simulink model "Rectifier"  (R2023b)
settings: Solver=VariableStepAuto  StartTime=0.0  StopTime=1  MaxStep=1e-4  RelTol=1e-4
values from neighbouring files (symbols this model uses):
  frequency_voltage1 = 60    [paramVals.mat]
  frequency_voltage2 = 60    [paramVals.mat]
  frequency_voltage3 = 60    [paramVals.mat]
  L = 0.2    [paramVals.mat]
  L1 = 0.005    [paramVals.mat]
  L2 = 0.005    [paramVals.mat]
  L3 = 0.005    [paramVals.mat]
  Load_Resistance_Ohm = 10    [paramVals.mat]
  peakAmplitude_voltage1 = 169.705627485    [paramVals.mat]
  peakAmplitude_voltage2 = 169.705627485    [paramVals.mat]
  peakAmplitude_voltage3 = 169.705627485    [paramVals.mat]
  phaseInDegree_voltage1 = 0    [paramVals.mat]
  phaseInDegree_voltage2 = -120    [paramVals.mat]
  phaseInDegree_voltage3 = 120    [paramVals.mat]
libraries: spsGroundLib x5, spsSeriesRLCBranchLib x5, spsDiodeLib x3, spsACVoltageSourceLib x3, spsCurrentMeasurementLib x1, spsVoltageMeasurementLib x1, spspowerguiLib x1
settings Model: Creator=The MathWorks, Inc.  LastModifiedBy=z004f2se
settings SolverCC: AlgebraicLoopSolver=TrustRegion
settings DataIOCC: ReturnWorkspaceOutputs=off  SignalLoggingName=sigsOut
settings OptimizationCC: BlockReduction=off  BooleanDataType=off  ExpressionDepthLimit=2147483647  InitFltsAndDblsToZero=on  EfficientMapNaN2IntZero=off  LifeSpan=inf
settings DebuggingCC: SaveWithParameterizedLinksMsg=none  UnderspecifiedInitializationDetection=Classic  MergeDetectMultiDrivingBlocksExec=none  CheckExecutionContextPreStartOutputMsg=on  SignalResolutionControl=TryResolveAllWithWarning  MultiTaskDSMMsg=warning  MultiTaskCondExecSysMsg=none  SigSpecEnsureSampleTimeMsg=none  FcnCallInpInsideContextMsg=warning  UnconnectedInputMsg=warning  UnconnectedOutputMsg=warning  UnconnectedLineMsg=warning  StateNameClashWarn=warning  SFUnexpectedBacktrackingDiag=warning  SFNoUnconditionalDefaultTransitionDiag=warning  SFExecutionAtInitializationDiag=none  ArithmeticOperatorsInVariantConditions=warning
settings HardwareCC: ProdBitPerPointer=32  ProdBitPerSizeT=32  ProdBitPerPtrDiffT=32  ProdLargestAtomicFloat=None  ProdIntDivRoundTo=Undefined  ProdEndianess=Unspecified  ProdWordSize=32  ProdHWDeviceType=32-bit Generic  TargetUnknown=on
settings ModelReferenceCC: EnableRefExpFcnMdlSchedulingChecks=on  PropagateSignalLabelsOutOfModel=off
settings SFSimCC: SimUseLocalCustomCode=off  CustomCodeUndefinedFunction=UseInterfaceOnly
settings RTWCC: RTWUseLocalCustomCode=off  DLArmComputeVersion=19.05
settings CodeAppCC: StateflowObjectComments=on
settings GRTTargetCC: TargetFcnLib=ansi_tfl_tmw.mat  TargetLangStandard=C89/C90 (ANSI)  CombineOutputUpdateFcns=off  GRTInterface=on
settings ConfigComp: CovMetricSettings=dw  CovSaveCumulativeToWorkspaceVar=on  CovSaveSingleToWorkspaceVar=on  CovExternalEMLEnable=off  CovSFcnEnable=off
settings SimscapeCC: SimscapeNormalizeSystem=off  SimscapeNominalValues={1, 'bar'; 1, 'cm^3/s'; 1, 'bar*kg/s'; 1, 'kJ/kg'; 1, 'kW'; }

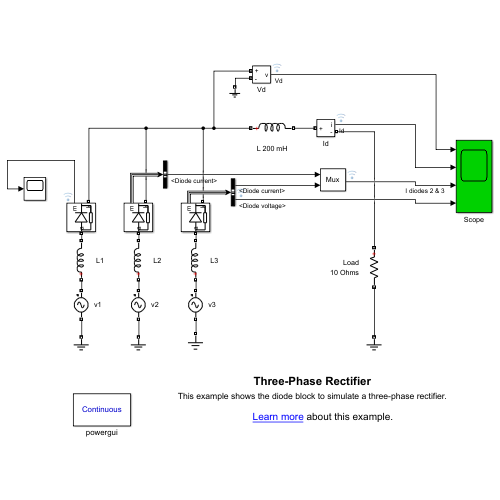
[thumbnail: Simulink's stored preview of the top-level diagram]
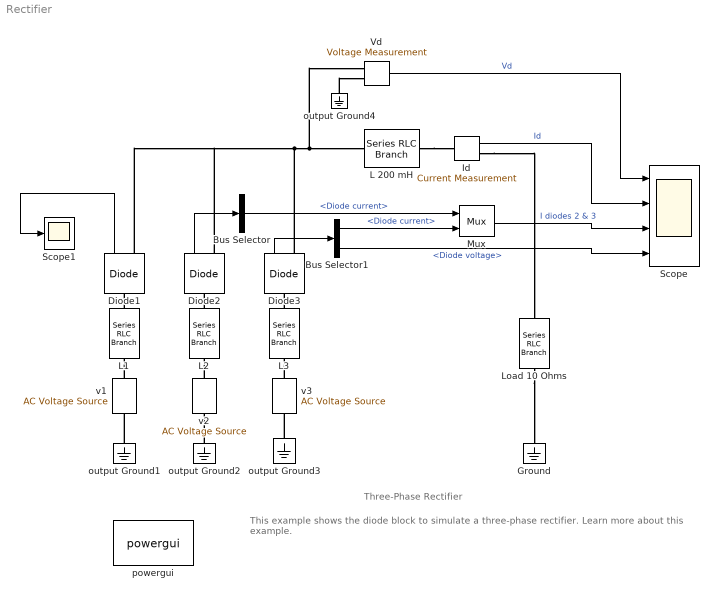
== system Rectifier ==
  note: Three-Phase Rectifier
  note: This example shows the diode block to simulate a three-phase rectifier.
      |
      | Learn more about this example.
  Bus Selector : BusSelector  OutputSignals=Diode current
  Bus Selector1 : BusSelector  OutputSignals=Diode current,Diode voltage
  Diode1 : spsDiodeLib/Diode  Ron=RonRes_Diode1  Lon=0  Vf=forwardVoltage_Diode1  IC=0  UseSnubber=off  Rs=snubberResmOhm_Diode1  Cs=snubberCapF_Diode1  Measurements=on
      settings: AttributesFormatString=\n
  Diode2 : spsDiodeLib/Diode  Ron=1e-2  Lon=0  Vf=0.8  IC=0  UseSnubber=off  Rs=1000  Cs=0.1e-6  Measurements=on
      settings: AttributesFormatString=\n
  Diode3 : spsDiodeLib/Diode  Ron=1e-2  Lon=0  Vf=0.8  IC=0  UseSnubber=off  Rs=1000  Cs=0.1e-6  Measurements=on
      settings: AttributesFormatString=\n
  Ground : spsGroundLib/Ground  LConnTagsString=a
  Id : spsCurrentMeasurementLib/Current Measurement  Tag=PoWeRsYsTeMmEaSuReMeNt  PhasorSimulation=off  OutputType=Magnitude  PSBequivalent=0
      settings: AttributesFormatString=\n
  L 200 mH : spsSeriesRLCBranchLib/Series RLC Branch  LConnTagsString=__new0  RConnTagsString=__new0  BranchType=L  Resistance=[]  Inductance=L  SetiL0=off  InitialCurrent=0  Capacitance=[]  Setx0=off  InitialVoltage=0  Measurements=None
  L1 : spsSeriesRLCBranchLib/Series RLC Branch  LConnTagsString=__new0  RConnTagsString=__new0  BranchType=L  Resistance=[]  Inductance=L1  SetiL0=off  InitialCurrent=0  Capacitance=[]  Setx0=off  InitialVoltage=0  Measurements=None
  L2 : spsSeriesRLCBranchLib/Series RLC Branch  LConnTagsString=__new0  RConnTagsString=__new0  BranchType=L  Resistance=[]  Inductance=L2  SetiL0=off  InitialCurrent=0  Capacitance=[]  Setx0=off  InitialVoltage=0  Measurements=None
  L3 : spsSeriesRLCBranchLib/Series RLC Branch  LConnTagsString=__new0  RConnTagsString=__new0  BranchType=L  Resistance=[]  Inductance=L3  SetiL0=off  InitialCurrent=0  Capacitance=[]  Setx0=off  InitialVoltage=0  Measurements=None
  Load 10 Ohms : spsSeriesRLCBranchLib/Series RLC Branch  LConnTagsString=__new0  RConnTagsString=__new0  BranchType=R  Resistance=Load_Resistance_Ohm  Inductance=[]  SetiL0=off  InitialCurrent=0  Capacitance=[]  Setx0=off  InitialVoltage=0  Measurements=None
  Mux : Mux  Inputs=2
  Scope : Scope  NumInputPorts=4
  Scope1 : Scope
  Vd : spsVoltageMeasurementLib/Voltage Measurement  Tag=PoWeRsYsTeMmEaSuReMeNt  PhasorSimulation=off  OutputType=Magnitude  PSBequivalent=0
  output Ground{1..4} (4 alike) : spsGroundLib/Ground  LConnTagsString=a
  powergui : spspowerguiLib/powergui  Priority=2  SimulationMode=Continuous  SampleTime=0  frequency=60  Iterations=50  frequencyindice=60  Pbase=100e6  ErrMax=1e-4  UnitsV=kV  UnitsW=MW  buscounter=0  FunctionMessages=off  echomessages=off  EnableUseOfTLC=off  CurrentSourceSwitches=off  DisableSnubberDevices=off  DisableRonSwitches=off  DisableVfSwitches=off  DisplayEquations=off  AutomaticDiscreteSolvers=off  SolverType=Tustin/Backward Euler (TBE)  Interpol=off  ExternalGateDelay=off  methode=off  Ts=100  x0status=blocks  SPID=on  SwTol=0  HookPort=off  NonlinearTolerance=1e-4  nMaxIteration=100  ContinueOnMaxIteration=off  RestoreLinks=warning  ResistiveCurrentMeasurement=off  Frange=[0:2:500]  Ylog=off  Xlog=on  ShowGrid=off  save=off  variable=ZData  structure=0  ZoomFFT=on  StartTime=0.0  cycles=1  DisplayStyle=1  fundamental=60  FreqAxis=off  MaxFrequency=1000  frequencyindicesteady=1  RmsSteady=1  display=off
  v1 : spsACVoltageSourceLib/AC Voltage Source  Description=source block  Amplitude=peakAmplitude_voltage1  Phase=phaseInDegree_voltage1  Frequency=frequency_voltage1  SampleTime=0  Measurements=None  BusType=swing  Pref=10e3  Qref=0  Qmin=-inf  Qmax=+inf
      settings: AttributesFormatString=\n
  v2 : spsACVoltageSourceLib/AC Voltage Source  Description=source block  Amplitude=peakAmplitude_voltage2  Phase=phaseInDegree_voltage2  Frequency=frequency_voltage2  SampleTime=0  Measurements=None  BusType=swing  Pref=10e3  Qref=0  Qmin=-inf  Qmax=+inf
      settings: AttributesFormatString=\n
  v3 : spsACVoltageSourceLib/AC Voltage Source  Description=source block  Amplitude=peakAmplitude_voltage3  Phase=phaseInDegree_voltage3  Frequency=frequency_voltage3  SampleTime=0  Measurements=None  BusType=swing  Pref=10e3  Qref=0  Qmin=-inf  Qmax=+inf
      settings: AttributesFormatString=\n
  wires:
  Bus Selector1/1 -> Mux/2  "<Diode current>"
  Mux/1 -> Scope/3  "I diodes 2 & 3"
  Bus Selector1/2 -> Scope/4  "<Diode voltage>"
  Diode2/1 -> Bus Selector/1
  Vd/1 -> Scope/1  "Vd"
  Id/1 -> Scope/2  "Id"
  Diode3/1 -> Bus Selector1/1
  Bus Selector/1 -> Mux/1  "<Diode current>"
  Diode1/1 -> Scope1/1
  connections:
  L 200 mH/RConn1 -- Id/LConn1
  Id/RConn1 -- Load 10 Ohms/LConn1
  Load 10 Ohms/RConn1 -- Ground/LConn1
  output Ground1/LConn1 -- v1/LConn1
  L1/RConn1 -- Diode1/LConn1
  v1/RConn1 -- L1/LConn1
  output Ground2/LConn1 -- v2/LConn1
  L2/RConn1 -- Diode2/LConn1
  v2/RConn1 -- L2/LConn1
  output Ground3/LConn1 -- v3/LConn1
  L3/RConn1 -- Diode3/LConn1
  v3/RConn1 -- L3/LConn1
  Diode1/RConn1 -- Diode2/RConn1 -- L 200 mH/LConn1 -- Vd/LConn1 -- Diode3/RConn1
  output Ground4/LConn1 -- Vd/LConn2
